simulink model "Demo1_P2A1"  (R2023a)
settings: Solver=VariableStepAuto  StartTime=0.0  StopTime=30  RelTol=1e-3
settings Model: Creator=rqouta  LastModifiedBy=rqouta

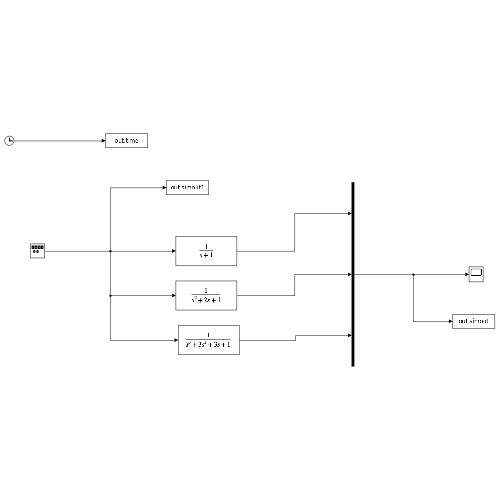
[thumbnail: Simulink's stored preview of the top-level diagram]
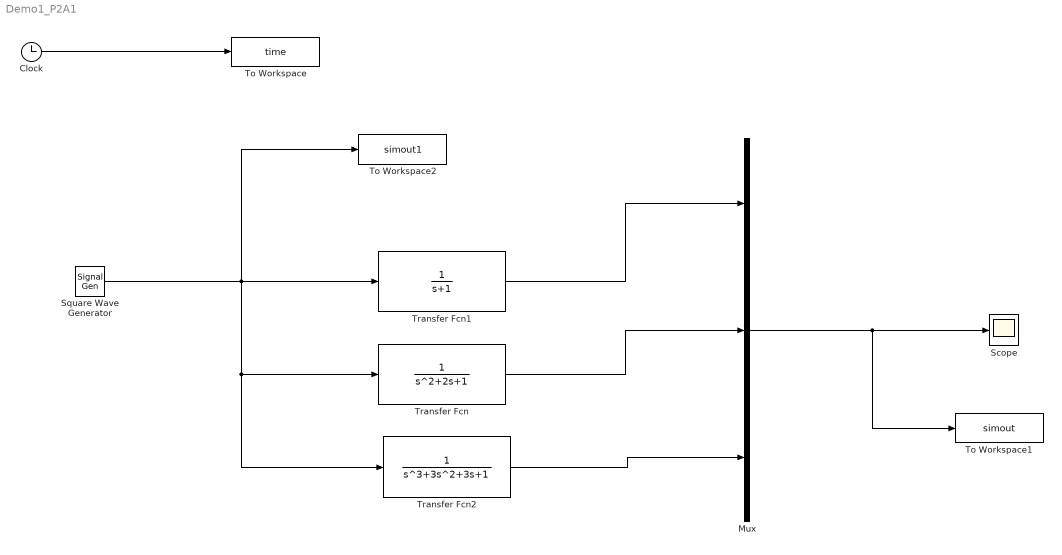
== system Demo1_P2A1 ==
  Clock : Clock
  Mux : Mux  Inputs=3
  Scope : Scope
  Square Wave Generator : SignalGenerator  WaveForm=square  Frequency=0.5  Units=rad/sec
  To Workspace : ToWorkspace  VariableName=time  SampleTime=-1
  To Workspace1 : ToWorkspace  VariableName=simout  SampleTime=-1
  To Workspace2 : ToWorkspace  VariableName=simout1  SampleTime=-1
  Transfer Fcn : TransferFcn
  Transfer Fcn1 : TransferFcn  Denominator=[1 1 ]
  Transfer Fcn2 : TransferFcn  Denominator=[1 3 3 1]
  wires:
  Clock/1 -> To Workspace/1
  Mux/1 -> To Workspace1/1, Scope/1
  Square Wave Generator/1 -> To Workspace2/1, Transfer Fcn1/1, Transfer Fcn/1, Transfer Fcn2/1
  Transfer Fcn2/1 -> Mux/3
  Transfer Fcn/1 -> Mux/2
  Transfer Fcn1/1 -> Mux/1
